simulink model "AC_motor_2_torque_control"  (R2024b)
settings: Solver=FixedStepAuto  StartTime=0.0  StopTime=Tsimulation  FixedStep=Ts  RelTol=1e-3
values from neighbouring files (symbols this model uses):
  J = 0.0226    [input_AIR80B4_2.m]    (also in input_AIR80B4_2_sc.m)
  Ki = 10    [input_AIR80B4_2.m]    (also in input_AIR80B4_2_sc.m)
  Kp = 10    [input_AIR80B4_2.m]    (also in input_AIR80B4_2_sc.m)
  P = 2    [input_AIR80B4_2.m]    (also in input_AIR80B4_2_sc.m)
  Rr = 1.274    [input_AIR80B4_2.m]    (also in input_AIR80B4_2_sc.m = Rr*((nturns_phase-fscnturns)/nturns_phase)^2)
  Rs = 3.523    [input_AIR80B4_2.m]    (also in input_AIR80B4_2_sc.m = Rs*((nturns_phase-fscnturns)/nturns_phase))
  Tlim = 11    [input_AIR80B4_2.m]    (also in input_AIR80B4_2_sc.m)
  Ts = 2e-5    (= 2e-05)    [input_AIR80B4_2.m]    (also in input_AIR80B4_2_sc.m)
  Tswrite = 0.24e-3    (= 0.00024)    [input_AIR80B4_2.m]    (also in input_AIR80B4_2_sc.m)
  Vdc = 460    [input_AIR80B4_2.m]    (also in input_AIR80B4_2_sc.m)
  wb = 2*pi*fb    (= 314.159265359)    [input_AIR80B4_2.m]    (also in input_AIR80B4_2_sc.m)
  Xlr = wb*Llr    (= 4.08407044967)    [input_AIR80B4_2.m]    (also in input_AIR80B4_2_sc.m)
  Xls = wb*Lls    (= 4.08407044967)    [input_AIR80B4_2.m]    (also in input_AIR80B4_2_sc.m)
  Xml = 1/(1/Xls+1/Xm+1/Xlr)    (= 2.00946288382)    [input_AIR80B4_2.m]    (also in input_AIR80B4_2_sc.m)
undefined symbols (not defined in the file or in its folder): DiscIntNeverNeededParam
libraries: simulink x2, spspowerguiLib x1
settings Model: Creator=rusla  LastModifiedBy=rusla

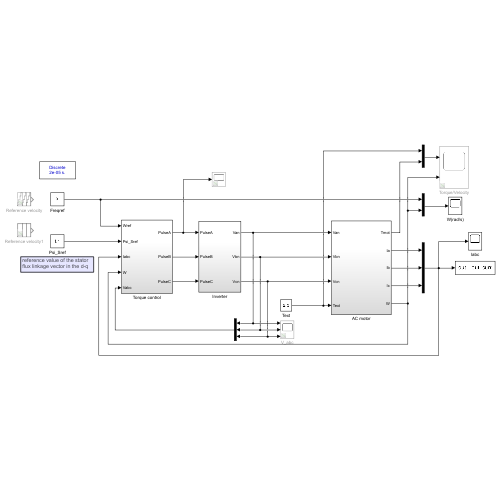
[thumbnail: Simulink's stored preview of the top-level diagram]
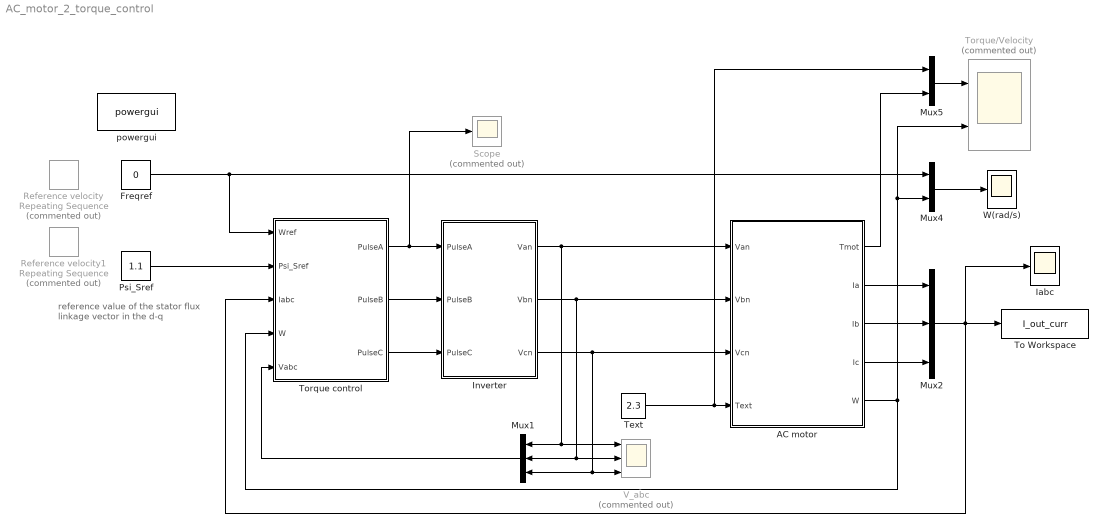
== system AC_motor_2_torque_control ==
  note: reference value of the stator
      | flux linkage vector in the d-q
  AC motor : Subsystem
  Freqref : Constant  Value=0
  Iabc : Scope
  Inverter : Subsystem
  Mux1 : Mux  Inputs=3
  Mux2 : Mux  Inputs=3
  Mux4 : Mux  Inputs=2
  Mux5 : Mux  Inputs=2
  Psi_Sref : Constant  Value=1.1
  Reference velocity : simulink/Sources/Repeating Sequence  Commented=on  rep_seq_t=[0 0.1 0.11 4 4.1 8 8.1 12 12.1 16]  rep_seq_y=[0 0 10 10 20 20 30 30 40 40]
  Reference velocity1 : simulink/Sources/Repeating Sequence  Commented=on  rep_seq_t=[0 0.1 0.11 10]  rep_seq_y=[0 0 2e-4 2e-4]
  Scope : Scope  Commented=on
  Text : Constant  Value=2.3
  To Workspace : ToWorkspace  VariableName=I_out_curr  SaveFormat=Structure With Time  SampleTime=Tswrite
  Torque control : Subsystem
  Torque/Velocity : Scope  Commented=on  NumInputPorts=2
  V_abc : Scope  Commented=on  NumInputPorts=3
  W(rad/s) : Scope
  powergui : spspowerguiLib/powergui  Priority=1  SimulationMode=Discrete  SampleTime=Ts  frequency=60  Iterations=50  frequencyindice=60  Pbase=100e6  ErrMax=1e-4  UnitsV=kV  UnitsW=MW  buscounter=0  FunctionMessages=off  echomessages=off  EnableUseOfTLC=off  CurrentSourceSwitches=off  DisableSnubberDevices=off  DisableRonSwitches=off  DisableVfSwitches=off  DisplayEquations=off  AutomaticDiscreteSolvers=off  SolverType=Tustin/Backward Euler (TBE)  Interpol=off  ExternalGateDelay=off  methode=off  Ts=100  x0status=blocks  SPID=on  SwTol=0  HookPort=off  NonlinearTolerance=1e-4  nMaxIteration=100  ContinueOnMaxIteration=off  RestoreLinks=warning  ResistiveCurrentMeasurement=off  Frange=[0:2:500]  Ylog=off  Xlog=on  ShowGrid=off  save=off  variable=ZData  structure=0  ZoomFFT=off  StartTime=0.0  cycles=1  DisplayStyle=1  fundamental=60  FreqAxis=off  MaxFrequency=1000  frequencyindicesteady=1  RmsSteady=1  display=off
  wires:
  Psi_Sref/1 -> Torque control/2(Psi_Sref)
  Freqref/1 -> Mux4/1, Torque control/1(Wref)
  Mux1/1 -> Torque control/5(Vabc)
  Inverter/1(Van) -> AC motor/1(Van), V_abc/1, Mux1/1
  Inverter/2(Vbn) -> AC motor/2(Vbn), V_abc/2, Mux1/2
  Inverter/3(Vcn) -> AC motor/3(Vcn), V_abc/3, Mux1/3
  Text/1 -> Mux5/1, AC motor/4(Text)
  Torque control/1(PulseA) -> Scope/1, Inverter/1(PulseA)
  Torque control/2(PulseB) -> Inverter/2(PulseB)
  Torque control/3(PulseC) -> Inverter/3(PulseC)
  AC motor/5(W) -> Torque control/4(W), Torque/Velocity/2, Mux4/2
  Mux2/1 -> To Workspace/1, Torque control/3(Iabc), Iabc/1
  AC motor/4(Ic) -> Mux2/3
  AC motor/3(Ib) -> Mux2/2
  AC motor/2(Ia) -> Mux2/1
  Mux4/1 -> W(rad/s)/1
  Mux5/1 -> Torque/Velocity/1
  AC motor/1(Tmot) -> Mux5/2

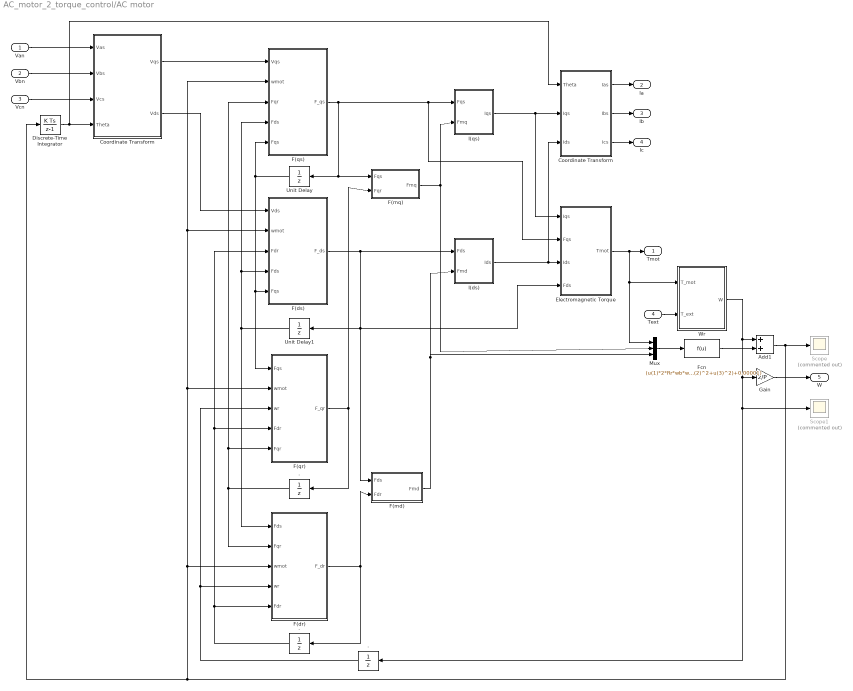
== system AC_motor_2_torque_control/AC motor ==
  Van : Inport
  Vbn : Inport  Port=2
  Vcn : Inport  Port=3
  Text : Inport  Port=4
  . : UnitDelay  SampleTime=Ts  HasFrameUpgradeWarning=on
  ". " : UnitDelay  SampleTime=Ts  HasFrameUpgradeWarning=on
  ".  " : UnitDelay  SampleTime=Ts  HasFrameUpgradeWarning=on
  Add1 : Sum
  Coordinate Transform : Subsystem
  "Coordinate Transform " : Subsystem
  Discrete-Time Integrator : DiscreteIntegrator  SampleTime=Ts  ICPrevOutput=DiscIntNeverNeededParam  ICPrevScaledInput=DiscIntNeverNeededParam
  Electromagnetic Torque : Subsystem
  F(dr) : Subsystem
  F(ds) : Subsystem
  F(md) : Subsystem
  F(mq) : Subsystem
  F(qr) : Subsystem
  F(qs) : Subsystem
  Fcn : Fcn  Expr=(u(1)*2*Rr*wb*wb)/(3*P*(u(2)^2+u(3)^2)+0.00001)
  Gain : Gain  Gain=2/P
  I(ds) : Subsystem
  I(qs) : Subsystem
  Mux : Mux  Inputs=3
  Scope : Scope  Commented=on
  Scope1 : Scope  Commented=on
  Unit Delay : UnitDelay  SampleTime=Ts  HasFrameUpgradeWarning=on
  Unit Delay1 : UnitDelay  SampleTime=Ts  HasFrameUpgradeWarning=on
  Wr : Subsystem
  Tmot : Outport
  Ia : Outport  Port=2
  Ib : Outport  Port=3
  Ic : Outport  Port=4
  W : Outport  Port=5
  wires:
  Gain/1 -> W/1
  Mux/1 -> Fcn/1
  Fcn/1 -> Add1/2
  F(md)/1(Fmd) -> I(ds)/2(Fmd), Mux/3
  ".  "/1 -> F(qr)/3(wr), F(dr)/4(wr)
  ". "/1 -> F(dr)/5(Fdr), F(qr)/4(Fdr), F(ds)/3(Fdr)
  ./1 -> F(dr)/2(Fqr), F(qs)/3(Fqr), F(qr)/5(Fqr)
  Unit Delay1/1 -> F(dr)/1(Fds), F(qs)/4(Fds), F(ds)/4(Fds)
  Unit Delay/1 -> F(qr)/1(Fqs), F(ds)/5(Fqs), F(qs)/5(Fqs)
  Add1/1 -> Scope/1, Discrete-Time Integrator/1, F(dr)/3(wmot), F(qr)/2(wmot), F(ds)/2(wmot), F(qs)/2("wmot ")
  Electromagnetic Torque/1(Tmot) -> Mux/1, Wr/1(T_mot), Tmot/1
  Text/1 -> Wr/2(T_ext)
  Discrete-Time Integrator/1 -> Coordinate Transform/1(Theta), "Coordinate Transform "/4(Theta)
  F(qs)/1(F_qs) -> Unit Delay/1, F(mq)/1(Fqs), I(qs)/1("Fqs "), Electromagnetic Torque/2(Fqs)
  F(qr)/1(F_qr) -> F(mq)/2(Fqr), ./1
  F(ds)/1(F_ds) -> Electromagnetic Torque/4(Fds), Unit Delay1/1, F(md)/1(Fds), I(ds)/1("Fds ")
  F(dr)/1(F_dr) -> F(md)/2(Fdr), ". "/1
  "Coordinate Transform "/1(Vqs) -> F(qs)/1(Vqs)
  Vbn/1 -> "Coordinate Transform "/2(Vbs)
  Vcn/1 -> "Coordinate Transform "/3(Vcs)
  "Coordinate Transform "/2(Vds) -> F(ds)/1(Vds)
  Van/1 -> "Coordinate Transform "/1(Vas)
  Wr/1(W) -> ".  "/1, Scope1/1, Gain/1, Add1/1
  I(qs)/1(Iqs) -> Coordinate Transform/2(Iqs), Electromagnetic Torque/1(Iqs)
  I(ds)/1(Ids) -> Coordinate Transform/3(Ids), Electromagnetic Torque/3(Ids)
  F(mq)/1(Fmq) -> Mux/2, I(qs)/2(Fmq)
  Coordinate Transform/1(Ias) -> Ia/1
  Coordinate Transform/2(Ibs) -> Ib/1
  Coordinate Transform/3(Ics) -> Ic/1

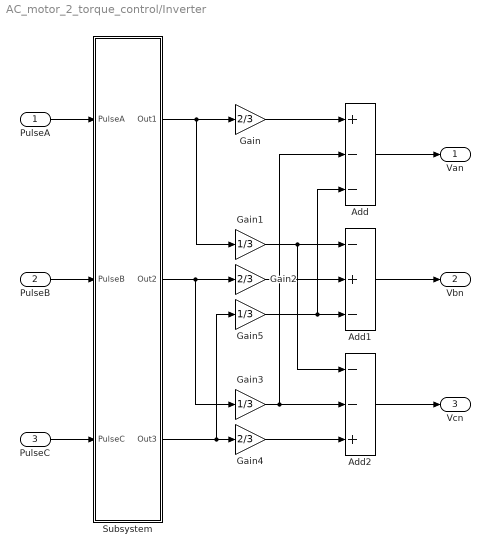
== system AC_motor_2_torque_control/Inverter ==
  PulseA : Inport
  PulseB : Inport  Port=2
  PulseC : Inport  Port=3
  Add : Sum  Inputs=+--
  Add1 : Sum  Inputs=-+-
  Add2 : Sum  Inputs=--+
  Gain : Gain  Gain=2/3
  Gain1 : Gain  Gain=1/3
  Gain2 : Gain  Gain=2/3
  Gain3 : Gain  Gain=1/3
  Gain4 : Gain  Gain=2/3
  Gain5 : Gain  Gain=1/3
  Subsystem : Subsystem
  Van : Outport
  Vbn : Outport  Port=2
  Vcn : Outport  Port=3
  wires:
  Gain1/1 -> Add1/1, Add2/1
  Gain2/1 -> Add1/2
  Gain/1 -> Add/1
  Gain5/1 -> Add1/3, Add/3
  Add1/1 -> Vbn/1
  Gain3/1 -> Add2/2, Add/2
  Add2/1 -> Vcn/1
  Add/1 -> Van/1
  Gain4/1 -> Add2/3
  Subsystem/1(Out1) -> Gain1/1, Gain/1
  Subsystem/3(Out3) -> Gain4/1, Gain5/1
  Subsystem/2(Out2) -> Gain3/1, Gain2/1
  PulseA/1 -> Subsystem/1(PulseA)
  PulseB/1 -> Subsystem/2(PulseB)
  PulseC/1 -> Subsystem/3(PulseC)

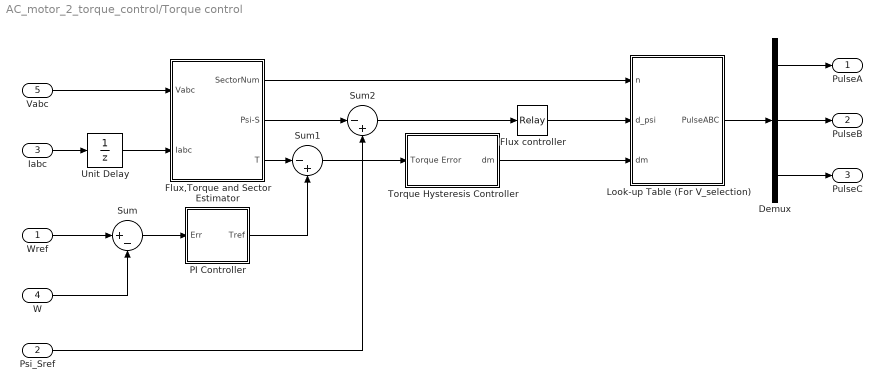
== system AC_motor_2_torque_control/Torque control ==
  Wref : Inport
  Psi_Sref : Inport  Port=2
  Iabc : Inport  Port=3
  W : Inport  Port=4
  Vabc : Inport  Port=5
  Demux : Demux  Outputs=3
  Flux controller : Relay  OnSwitchValue=0.02  OffSwitchValue=-0.02
  Flux,Torque and Sector Estimator : Subsystem
  Look-up Table (For V_selection) : MATLAB Function  TreatAsAtomicUnit=on
  PI Controller : Subsystem
  Sum : Sum  Inputs=|+-
  Sum1 : Sum  Inputs=|-+
  Sum2 : Sum  Inputs=|-+
  Torque Hysteresis Controller : Subsystem
  Unit Delay : UnitDelay  SampleTime=-1  HasFrameUpgradeWarning=on
  PulseA : Outport
  PulseB : Outport  Port=2
  PulseC : Outport  Port=3
  wires:
  Look-up Table (For V_selection)/1(PulseABC) -> Demux/1
  Vabc/1 -> Flux,Torque and Sector Estimator/1(Vabc)
  Demux/2 -> PulseB/1
  Demux/1 -> PulseA/1
  Unit Delay/1 -> Flux,Torque and Sector Estimator/2(Iabc)
  Demux/3 -> PulseC/1
  Wref/1 -> Sum/1
  Flux,Torque and Sector Estimator/3(T) -> Sum1/1
  Iabc/1 -> Unit Delay/1
  Sum1/1 -> Torque Hysteresis Controller/1(Torque Error)
  Sum/1 -> PI Controller/1(Err)
  Psi_Sref/1 -> Sum2/2
  Torque Hysteresis Controller/1(dm) -> Look-up Table (For V_selection)/3(dm)
  W/1 -> Sum/2
  Flux,Torque and Sector Estimator/1(SectorNum) -> Look-up Table (For V_selection)/1(n)
  Sum2/1 -> Flux controller/1
  Flux,Torque and Sector Estimator/2(Psi-S) -> Sum2/1
  Flux controller/1 -> Look-up Table (For V_selection)/2(d_psi)
  PI Controller/1(Tref) -> Sum1/2

== system AC_motor_2_torque_control/AC motor/Coordinate Transform ==
  Theta : Inport
  Iqs : Inport  Port=2
  Ids : Inport  Port=3
  Inverse Clark Transform : Subsystem
  Inverse Park Transform : Subsystem
  Ias : Outport
  Ibs : Outport  Port=2
  Ics : Outport  Port=3
  wires:
  Ids/1 -> Inverse Park Transform/2(Ids)
  Inverse Park Transform/2(I(qss)) -> Inverse Clark Transform/2(Iqss)
  Iqs/1 -> Inverse Park Transform/3(Iqs)
  Theta/1 -> Inverse Park Transform/1(Theta)
  Inverse Park Transform/1(I(dss)) -> Inverse Clark Transform/1(Idss)
  Inverse Clark Transform/2(Ibs) -> Ibs/1
  Inverse Clark Transform/1(Ias) -> Ias/1
  Inverse Clark Transform/3(Ics) -> Ics/1

== system AC_motor_2_torque_control/AC motor/Coordinate Transform  ==
  Vas : Inport
  Vbs : Inport  Port=2
  Vcs : Inport  Port=3
  Theta : Inport  Port=4
  Clark transform (betta inverted) 3 phase to 2 phase : Subsystem
  Park transform : Subsystem
  Vqs : Outport
  Vds : Outport  Port=2
  wires:
  Clark transform (betta inverted) 3 phase to 2 phase/1(Valpha) -> Park transform/1(Valpha)
  Clark transform (betta inverted) 3 phase to 2 phase/2(Vbetta) -> Park transform/2(Vbetta)
  Park transform/2("Vqs ") -> Vqs/1
  Theta/1 -> Park transform/3("Theta( e) (in rad.) ")
  Park transform/1(Vds) -> Vds/1
  Vbs/1 -> Clark transform (betta inverted) 3 phase to 2 phase/2(Vbs)
  Vcs/1 -> Clark transform (betta inverted) 3 phase to 2 phase/3(Vcs)
  Vas/1 -> Clark transform (betta inverted) 3 phase to 2 phase/1(Vas)

== system AC_motor_2_torque_control/AC motor/Electromagnetic Torque ==
  Iqs : Inport
  Fqs : Inport  Port=2
  Ids : Inport  Port=3
  Fds : Inport  Port=4
  Add : Sum  Inputs=+-
  Gain : Gain  Gain=(3*P)/(4*wb)
  Product : Product
  Product1 : Product
  Tmot : Outport
  wires:
  Product1/1 -> Add/2
  Add/1 -> Gain/1
  Product/1 -> Add/1
  Iqs/1 -> Product/2
  Ids/1 -> Product1/2
  Fqs/1 -> Product1/1
  Fds/1 -> Product/1
  Gain/1 -> Tmot/1

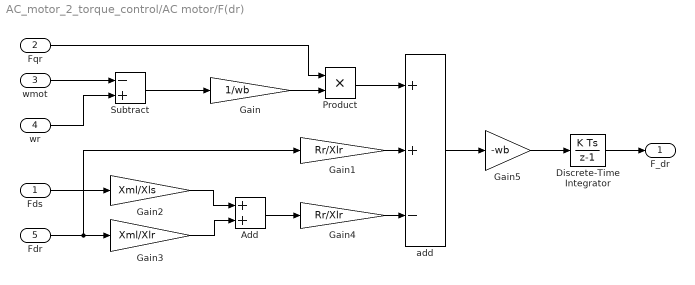
== system AC_motor_2_torque_control/AC motor/F(dr) ==
  Fds : Inport
  Fqr : Inport  Port=2
  wmot : Inport  Port=3
  wr : Inport  Port=4
  Fdr : Inport  Port=5
  Add : Sum
  Discrete-Time Integrator : DiscreteIntegrator  SampleTime=Ts  ICPrevOutput=DiscIntNeverNeededParam  ICPrevScaledInput=DiscIntNeverNeededParam
  Gain : Gain  Gain=1/wb
  Gain1 : Gain  Gain=Rr/Xlr
  Gain2 : Gain  Gain=Xml/Xls
  Gain3 : Gain  Gain=Xml/Xlr
  Gain4 : Gain  Gain=Rr/Xlr
  Gain5 : Gain  Gain=-wb
  Product : Product
  Subtract : Sum  Inputs=-+
  add : Sum  Inputs=++-
  F_dr : Outport
  wires:
  Product/1 -> add/1
  Fqr/1 -> Product/1
  Fdr/1 -> Gain1/1, Gain3/1
  Gain4/1 -> add/3
  Gain1/1 -> add/2
  wr/1 -> Subtract/2
  Gain/1 -> Product/2
  Gain3/1 -> Add/2
  Gain2/1 -> Add/1
  Fds/1 -> Gain2/1
  Add/1 -> Gain4/1
  Subtract/1 -> Gain/1
  wmot/1 -> Subtract/1
  add/1 -> Gain5/1
  Gain5/1 -> Discrete-Time Integrator/1
  Discrete-Time Integrator/1 -> F_dr/1

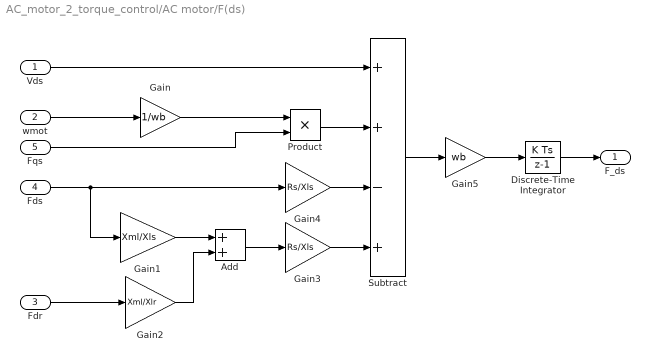
== system AC_motor_2_torque_control/AC motor/F(ds) ==
  Vds : Inport
  wmot : Inport  Port=2
  Fdr : Inport  Port=3
  Fds : Inport  Port=4
  Fqs : Inport  Port=5
  Add : Sum
  Discrete-Time Integrator : DiscreteIntegrator  SampleTime=Ts  ICPrevOutput=DiscIntNeverNeededParam  ICPrevScaledInput=DiscIntNeverNeededParam
  Gain : Gain  Gain=1/wb
  Gain1 : Gain  Gain=Xml/Xls
  Gain2 : Gain  Gain=Xml/Xlr
  Gain3 : Gain  Gain=Rs/Xls
  Gain4 : Gain  Gain=Rs/Xls
  Gain5 : Gain  Gain=wb
  Product : Product
  Subtract : Sum  Inputs=++-+
  F_ds : Outport
  wires:
  wmot/1 -> Gain/1
  Fdr/1 -> Gain2/1
  Gain1/1 -> Add/1
  Fds/1 -> Gain1/1, Gain4/1
  Gain4/1 -> Subtract/3
  Gain3/1 -> Subtract/4
  Add/1 -> Gain3/1
  Fqs/1 -> Product/2
  Product/1 -> Subtract/2
  Gain5/1 -> Discrete-Time Integrator/1
  Subtract/1 -> Gain5/1
  Discrete-Time Integrator/1 -> F_ds/1
  Gain2/1 -> Add/2
  Vds/1 -> Subtract/1
  Gain/1 -> Product/1

== system AC_motor_2_torque_control/AC motor/F(md) ==
  Fds : Inport
  Fdr : Inport  Port=2
  Add : Sum
  Gain1 : Gain  Gain=Xml/Xls
  Gain2 : Gain  Gain=Xml/Xlr
  Fmd : Outport
  wires:
  Gain1/1 -> Add/1
  Gain2/1 -> Add/2
  Fdr/1 -> Gain2/1
  Fds/1 -> Gain1/1
  Add/1 -> Fmd/1

== system AC_motor_2_torque_control/AC motor/F(mq) ==
  Fqs : Inport
  Fqr : Inport  Port=2
  Add : Sum
  Gain1 : Gain  Gain=Xml/Xls
  Gain2 : Gain  Gain=Xml/Xlr
  Fmq : Outport
  wires:
  Add/1 -> Fmq/1
  Fqs/1 -> Gain1/1
  Fqr/1 -> Gain2/1
  Gain2/1 -> Add/2
  Gain1/1 -> Add/1

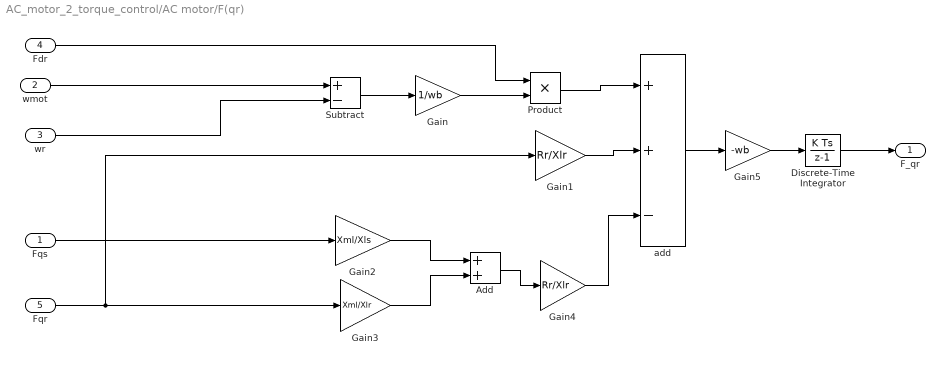
== system AC_motor_2_torque_control/AC motor/F(qr) ==
  Fqs : Inport
  wmot : Inport  Port=2
  wr : Inport  Port=3
  Fdr : Inport  Port=4
  Fqr : Inport  Port=5
  Add : Sum
  Discrete-Time Integrator : DiscreteIntegrator  SampleTime=Ts  ICPrevOutput=DiscIntNeverNeededParam  ICPrevScaledInput=DiscIntNeverNeededParam
  Gain : Gain  Gain=1/wb
  Gain1 : Gain  Gain=Rr/Xlr
  Gain2 : Gain  Gain=Xml/Xls
  Gain3 : Gain  Gain=Xml/Xlr
  Gain4 : Gain  Gain=Rr/Xlr
  Gain5 : Gain  Gain=-wb
  Product : Product
  Subtract : Sum  Inputs=+-
  add : Sum  Inputs=++-
  F_qr : Outport
  wires:
  Discrete-Time Integrator/1 -> F_qr/1
  Gain5/1 -> Discrete-Time Integrator/1
  add/1 -> Gain5/1
  wmot/1 -> Subtract/1
  Subtract/1 -> Gain/1
  Add/1 -> Gain4/1
  Fqs/1 -> Gain2/1
  Gain2/1 -> Add/1
  Gain3/1 -> Add/2
  Gain/1 -> Product/2
  wr/1 -> Subtract/2
  Gain1/1 -> add/2
  Gain4/1 -> add/3
  Fqr/1 -> Gain3/1, Gain1/1
  Fdr/1 -> Product/1
  Product/1 -> add/1

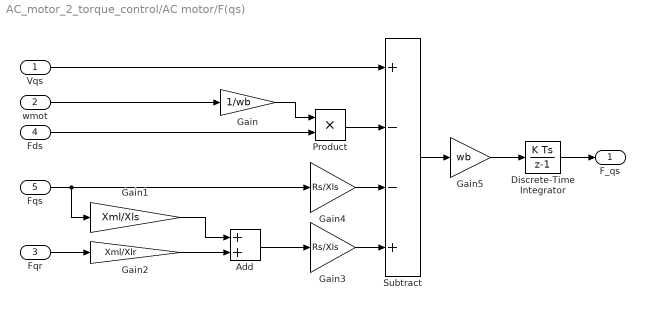
== system AC_motor_2_torque_control/AC motor/F(qs) ==
  Vqs : Inport
  "wmot " : Inport  Port=2
  Fqr : Inport  Port=3
  Fds : Inport  Port=4
  Fqs : Inport  Port=5
  Add : Sum
  Discrete-Time Integrator : DiscreteIntegrator  SampleTime=Ts  ICPrevOutput=DiscIntNeverNeededParam  ICPrevScaledInput=DiscIntNeverNeededParam
  Gain : Gain  Gain=1/wb
  Gain1 : Gain  Gain=Xml/Xls
  Gain2 : Gain  Gain=Xml/Xlr
  Gain3 : Gain  Gain=Rs/Xls
  Gain4 : Gain  Gain=Rs/Xls
  Gain5 : Gain  Gain=wb
  Product : Product
  Subtract : Sum  Inputs=+--+
  F_qs : Outport
  wires:
  Gain/1 -> Product/1
  Vqs/1 -> Subtract/1
  Gain2/1 -> Add/2
  Discrete-Time Integrator/1 -> F_qs/1
  Subtract/1 -> Gain5/1
  Gain5/1 -> Discrete-Time Integrator/1
  Product/1 -> Subtract/2
  Fds/1 -> Product/2
  Add/1 -> Gain3/1
  Gain3/1 -> Subtract/4
  Gain4/1 -> Subtract/3
  Fqs/1 -> Gain1/1, Gain4/1
  Gain1/1 -> Add/1
  Fqr/1 -> Gain2/1
  "wmot "/1 -> Gain/1

== system AC_motor_2_torque_control/AC motor/I(ds) ==
  "Fds " : Inport
  Fmd : Inport  Port=2
  Gain : Gain  Gain=1/Xls
  Subtract : Sum  Inputs=+-
  Ids : Outport
  wires:
  Fmd/1 -> Subtract/2
  "Fds "/1 -> Subtract/1
  Subtract/1 -> Gain/1
  Gain/1 -> Ids/1

== system AC_motor_2_torque_control/AC motor/I(qs) ==
  "Fqs " : Inport
  Fmq : Inport  Port=2
  Gain : Gain  Gain=1/Xls
  Subtract : Sum  Inputs=+-
  Iqs : Outport
  wires:
  Gain/1 -> Iqs/1
  Subtract/1 -> Gain/1
  "Fqs "/1 -> Subtract/1
  Fmq/1 -> Subtract/2

== system AC_motor_2_torque_control/AC motor/Wr ==
  T_mot : Inport
  T_ext : Inport  Port=2
  Add : Sum  Inputs=+-
  Discrete-Time Integrator : DiscreteIntegrator  gainval=Ktorquegain  SampleTime=Ts  ICPrevOutput=DiscIntNeverNeededParam  ICPrevScaledInput=DiscIntNeverNeededParam
  Gain : Gain  Gain=P/(2*J)
  W : Outport
  wires:
  T_mot/1 -> Add/1
  T_ext/1 -> Add/2
  Add/1 -> Gain/1
  Gain/1 -> Discrete-Time Integrator/1
  Discrete-Time Integrator/1 -> W/1

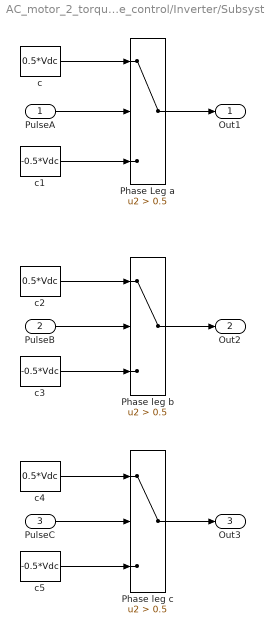
== system AC_motor_2_torque_control/Inverter/Subsystem ==
  PulseA : Inport
  PulseB : Inport  Port=2
  PulseC : Inport  Port=3
  Phase Leg a : Switch  Criteria=u2 > Threshold  Threshold=0.5  SaturateOnIntegerOverflow=off  InputSameDT=off
  Phase leg b : Switch  Criteria=u2 > Threshold  Threshold=0.5  SaturateOnIntegerOverflow=off  InputSameDT=off
  "Phase leg c " : Switch  Criteria=u2 > Threshold  Threshold=0.5  SaturateOnIntegerOverflow=off  InputSameDT=off
  c : Constant  Value=0.5*Vdc
  c1 : Constant  Value=-0.5*Vdc
  c2 : Constant  Value=0.5*Vdc
  c3 : Constant  Value=-0.5*Vdc
  c4 : Constant  Value=0.5*Vdc
  c5 : Constant  Value=-0.5*Vdc
  Out1 : Outport
  Out2 : Outport  Port=2
  Out3 : Outport  Port=3
  wires:
  "Phase leg c "/1 -> Out3/1
  c5/1 -> "Phase leg c "/3
  c3/1 -> Phase leg b/3
  c/1 -> Phase Leg a/1
  Phase Leg a/1 -> Out1/1
  Phase leg b/1 -> Out2/1
  c4/1 -> "Phase leg c "/1
  PulseB/1 -> Phase leg b/2
  PulseA/1 -> Phase Leg a/2
  PulseC/1 -> "Phase leg c "/2
  c1/1 -> Phase Leg a/3
  c2/1 -> Phase leg b/1

== system AC_motor_2_torque_control/Torque control/Flux,Torque and Sector Estimator ==
  Vabc : Inport
  Iabc : Inport  Port=2
  Flux and Torque Estimator : Subsystem
  Scope : Scope  Commented=on
  Sector Estimation : MATLAB Function  TreatAsAtomicUnit=on
  SectorNum : Outport
  Psi-S : Outport  Port=2
  T : Outport  Port=3
  wires:
  Iabc/1 -> Flux and Torque Estimator/2(Iabc)
  Vabc/1 -> Flux and Torque Estimator/1(V_abc)
  Flux and Torque Estimator/4(PsiBeta) -> Sector Estimation/2(PsiBeta)
  Flux and Torque Estimator/3(PsiAlpha) -> Sector Estimation/1(PsiAlpha)
  Sector Estimation/1(n) -> SectorNum/1
  Flux and Torque Estimator/1(Psi_S) -> Psi-S/1
  Flux and Torque Estimator/2(TransientTorque) -> T/1
  Sector Estimation/2(angl) -> Scope/1

== system AC_motor_2_torque_control/Torque control/PI Controller ==
  Err : Inport
  "Integrator " : DiscreteIntegrator  SampleTime=Ts  LimitOutput=on  UpperSaturationLimit=Tlim  LowerSaturationLimit=-Tlim  ICPrevOutput=DiscIntNeverNeededParam  ICPrevScaledInput=DiscIntNeverNeededParam
  Ki : Gain  Gain=Ki
  Kp : Gain  Gain=Kp
  Saturation : Saturate  UpperLimit=Tlim  LowerLimit=-Tlim
  Sum1 : Sum  Inputs=|++
  Tref : Outport
  wires:
  Saturation/1 -> Tref/1
  Sum1/1 -> Saturation/1
  "Integrator "/1 -> Sum1/2
  Kp/1 -> Sum1/1
  Ki/1 -> "Integrator "/1
  Err/1 -> Kp/1, Ki/1

== system AC_motor_2_torque_control/Torque control/Torque Hysteresis Controller ==
  Torque Error : Inport
  Add : Sum
  Flux controller1 : Relay  OnSwitchValue=0.2  OffSwitchValue=0
  Flux controller2 : Relay  OnSwitchValue=0  OffSwitchValue=-0.2  OnOutputValue=0  OffOutputValue=-1
  dm : Outport
  wires:
  Torque Error/1 -> Flux controller1/1, Flux controller2/1
  Flux controller1/1 -> Add/1
  Flux controller2/1 -> Add/2
  Add/1 -> dm/1

== system AC_motor_2_torque_control/AC motor/Coordinate Transform/Inverse Clark Transform ==
  Idss : Inport
  Iqss : Inport  Port=2
  Add : Sum
  Add1 : Sum
  Gain : Gain  Gain=-0.5
  Gain1 : Gain  Gain=-sqrt(3)/2
  Gain2 : Gain  Gain=-0.5
  Gain3 : Gain  Gain=sqrt(3)/2
  Ias : Outport
  Ibs : Outport  Port=2
  Ics : Outport  Port=3
  wires:
  Iqss/1 -> Gain/1, Ias/1, Gain2/1
  Idss/1 -> Gain1/1, Gain3/1
  Gain/1 -> Add/1
  Gain1/1 -> Add/2
  Add1/1 -> Ics/1
  Gain2/1 -> Add1/1
  Add/1 -> Ibs/1
  Gain3/1 -> Add1/2

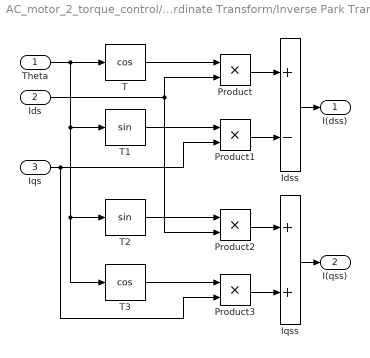
== system AC_motor_2_torque_control/AC motor/Coordinate Transform/Inverse Park Transform ==
  Theta : Inport
  Ids : Inport  Port=2
  Iqs : Inport  Port=3
  Idss : Sum  Inputs=+-
  Iqss : Sum
  Product{,1..3} (4 alike) : Product
  T : Trigonometry  Operator=cos
  T1 : Trigonometry
  T2 : Trigonometry
  T3 : Trigonometry  Operator=cos
  I(dss) : Outport
  I(qss) : Outport  Port=2
  wires:
  T3/1 -> Product3/1
  Product2/1 -> Iqss/1
  Ids/1 -> Product2/2, Product/2
  Theta/1 -> T1/1, T3/1, T2/1, T/1
  Product3/1 -> Iqss/2
  Iqs/1 -> Product3/2, Product1/2
  T2/1 -> Product2/1
  T1/1 -> Product1/1
  Iqss/1 -> I(qss)/1
  Idss/1 -> I(dss)/1
  Product1/1 -> Idss/2
  Product/1 -> Idss/1
  T/1 -> Product/1

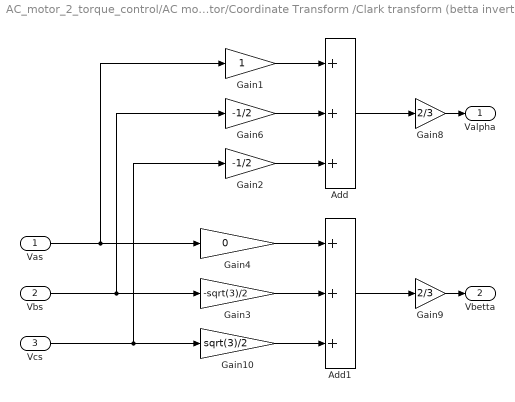
== system AC_motor_2_torque_control/AC motor/Coordinate Transform /Clark transform (betta inverted) 3 phase to 2 phase ==
  Vas : Inport
  Vbs : Inport  Port=2
  Vcs : Inport  Port=3
  Add : Sum  Inputs=+++
  Add1 : Sum  Inputs=+++
  Gain1 : Gain
  Gain10 : Gain  Gain=sqrt(3)/2
  Gain2 : Gain  Gain=-1/2
  Gain3 : Gain  Gain=-sqrt(3)/2
  Gain4 : Gain  Gain=0
  Gain6 : Gain  Gain=-1/2
  Gain8 : Gain  Gain=2/3
  Gain9 : Gain  Gain=2/3
  Valpha : Outport
  Vbetta : Outport  Port=2
  wires:
  Gain2/1 -> Add/3
  Gain9/1 -> Vbetta/1
  Gain8/1 -> Valpha/1
  Add1/1 -> Gain9/1
  Add/1 -> Gain8/1
  Gain6/1 -> Add/2
  Gain1/1 -> Add/1
  Gain4/1 -> Add1/1
  Gain3/1 -> Add1/2
  Vcs/1 -> Gain10/1, Gain2/1
  Gain10/1 -> Add1/3
  Vas/1 -> Gain4/1, Gain1/1
  Vbs/1 -> Gain6/1, Gain3/1

== system AC_motor_2_torque_control/AC motor/Coordinate Transform /Park transform ==
  Valpha : Inport
  Vbetta : Inport  Port=2
  "Theta( e) (in rad.) " : Inport  Port=3
  Add : Sum
  Add2 : Sum  Inputs=+-
  Product{,1..2,4} (4 alike) : Product
  t : Trigonometry  Operator=cos
  t1 : Trigonometry
  t2 : Trigonometry  Operator=cos
  t3 : Trigonometry
  Vds : Outport
  "Vqs " : Outport  Port=2
  wires:
  Valpha/1 -> Product4/1, Product1/1
  Product2/1 -> Add2/2
  t3/1 -> Product2/2
  Product4/1 -> Add2/1
  t2/1 -> Product4/2
  Product1/1 -> Add/2
  t1/1 -> Product1/2
  Product/1 -> Add/1
  Add2/1 -> "Vqs "/1
  Add/1 -> Vds/1
  "Theta( e) (in rad.) "/1 -> t3/1, t2/1, t/1, t1/1
  Vbetta/1 -> Product2/1, Product/1
  t/1 -> Product/2

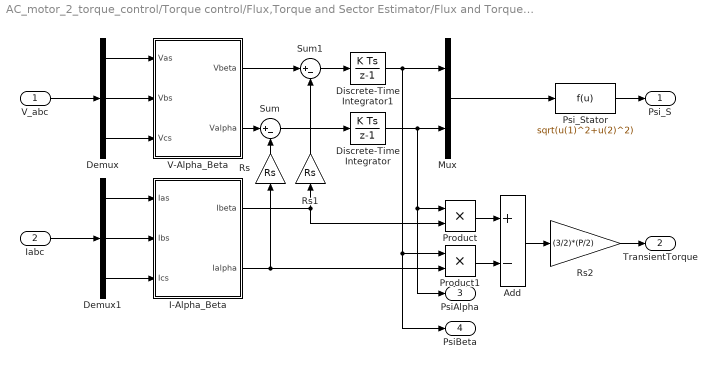
== system AC_motor_2_torque_control/Torque control/Flux,Torque and Sector Estimator/Flux and Torque Estimator ==
  V_abc : Inport
  Iabc : Inport  Port=2
  Add : Sum  Inputs=+-
  Demux : Demux  Outputs=3
  Demux1 : Demux  Outputs=3
  Discrete-Time Integrator : DiscreteIntegrator  SampleTime=Ts  ICPrevOutput=DiscIntNeverNeededParam  ICPrevScaledInput=DiscIntNeverNeededParam
  Discrete-Time Integrator1 : DiscreteIntegrator  SampleTime=Ts  ICPrevOutput=DiscIntNeverNeededParam  ICPrevScaledInput=DiscIntNeverNeededParam
  I-Alpha_Beta : Subsystem
  Mux : Mux  Inputs=2
  Product : Product
  Product1 : Product
  Psi_Stator : Fcn  Expr=sqrt(u(1)^2+u(2)^2)
  Rs : Gain  Gain=Rs
  Rs1 : Gain  Gain=Rs
  Rs2 : Gain  Gain=(3/2)*(P/2)
  Sum : Sum  Inputs=|+-
  Sum1 : Sum  Inputs=|+-
  V-Alpha_Beta : Subsystem
  Psi_S : Outport
  TransientTorque : Outport  Port=2
  PsiAlpha : Outport  Port=3
  PsiBeta : Outport  Port=4
  wires:
  Discrete-Time Integrator1/1 -> PsiBeta/1, Product1/1, Mux/1
  Rs2/1 -> TransientTorque/1
  Psi_Stator/1 -> Psi_S/1
  Add/1 -> Rs2/1
  Product1/1 -> Add/2
  Product/1 -> Add/1
  Discrete-Time Integrator/1 -> Product/1, PsiAlpha/1, Mux/2
  Mux/1 -> Psi_Stator/1
  Sum1/1 -> Discrete-Time Integrator1/1
  Rs1/1 -> Sum1/2
  Sum/1 -> Discrete-Time Integrator/1
  Rs/1 -> Sum/2
  Demux/2 -> V-Alpha_Beta/2(Vbs)
  Demux/1 -> V-Alpha_Beta/1(Vas)
  V_abc/1 -> Demux/1
  Demux/3 -> V-Alpha_Beta/3(Vcs)
  I-Alpha_Beta/2(Ialpha) -> Rs/1, Product1/2
  I-Alpha_Beta/1(Ibeta) -> Rs1/1, Product/2
  V-Alpha_Beta/1(Vbeta) -> Sum1/1
  V-Alpha_Beta/2(Valpha) -> Sum/1
  Demux1/2 -> I-Alpha_Beta/2(Ibs)
  Demux1/3 -> I-Alpha_Beta/3(Ics)
  Demux1/1 -> I-Alpha_Beta/1(Ias)
  Iabc/1 -> Demux1/1

== system AC_motor_2_torque_control/Torque control/Flux,Torque and Sector Estimator/Flux and Torque Estimator/I-Alpha_Beta ==
  Ias : Inport
  Ibs : Inport  Port=2
  Ics : Inport  Port=3
  Add : Sum  Inputs=+++
  Add1 : Sum  Inputs=+++
  Gain : Gain  Gain=0
  Gain1 : Gain  Gain=sqrt(3)/2
  Gain2 : Gain  Gain=-sqrt(3)/2
  Gain3 : Gain
  Gain4 : Gain  Gain=-1/2
  Gain5 : Gain  Gain=-1/2
  Gain8 : Gain  Gain=2/3
  Gain9 : Gain  Gain=2/3
  Ibeta : Outport
  Ialpha : Outport  Port=2
  wires:
  Ibs/1 -> Gain1/1, Gain4/1
  Ias/1 -> Gain/1, Gain3/1
  Gain5/1 -> Add1/3
  Ics/1 -> Gain5/1, Gain2/1
  Gain4/1 -> Add1/2
  Gain3/1 -> Add1/1
  Gain/1 -> Add/1
  Gain1/1 -> Add/2
  Add/1 -> Gain8/1
  Add1/1 -> Gain9/1
  Gain8/1 -> Ibeta/1
  Gain9/1 -> Ialpha/1
  Gain2/1 -> Add/3

== system AC_motor_2_torque_control/Torque control/Flux,Torque and Sector Estimator/Flux and Torque Estimator/V-Alpha_Beta ==
  Vas : Inport
  Vbs : Inport  Port=2
  Vcs : Inport  Port=3
  Add : Sum  Inputs=+++
  Add1 : Sum  Inputs=+++
  Gain : Gain  Gain=0
  Gain1 : Gain  Gain=sqrt(3)/2
  Gain2 : Gain  Gain=-sqrt(3)/2
  Gain3 : Gain
  Gain4 : Gain  Gain=-1/2
  Gain5 : Gain  Gain=-1/2
  Gain8 : Gain  Gain=2/3
  Gain9 : Gain  Gain=2/3
  Vbeta : Outport
  Valpha : Outport  Port=2
  wires:
  Gain2/1 -> Add/3
  Gain9/1 -> Valpha/1
  Gain8/1 -> Vbeta/1
  Add1/1 -> Gain9/1
  Add/1 -> Gain8/1
  Gain1/1 -> Add/2
  Gain/1 -> Add/1
  Gain3/1 -> Add1/1
  Gain4/1 -> Add1/2
  Vcs/1 -> Gain5/1, Gain2/1
  Gain5/1 -> Add1/3
  Vas/1 -> Gain/1, Gain3/1
  Vbs/1 -> Gain1/1, Gain4/1

== matlab function AC_motor_2_torque_control/Torque control/Look-up Table (For V_selection) ==
  data: n input; d_psi input; PulseABC output; dm input
function PulseABC=V_selection(n,d_psi,dm)
v=0;
%SECTOR 1 :
if(n==1)&&(d_psi==1)&&(dm==1)
    v=2;
elseif(n==1)&&(d_psi==1)&&(dm==0)
    v=7;
elseif(n==1)&&(d_psi==1)&&(dm==-1)
    v=6;
elseif(n==1)&&(d_psi==0)&&(dm==1)
    v=3;
elseif(n==1)&&(d_psi==0)&&(dm==0)
    v=0;
elseif(n==1)&&(d_psi==0)&&(dm==-1)
    v=5;
%SECTOR 2 :
elseif(n==2)&&(d_psi==1)&&(dm==1)
    v=3;
elseif(n==2)&&(d_psi==1)&&(dm==0)
    v=0;
elseif(n==2)&&(d_psi==1)&&(dm==-1)
    v=1;
elseif(n==2)&&(d_psi==0)&&(dm==1)
    v=4;
elseif(n==2)&&(d_psi==0)&&(dm==0)
    v=7;
elseif(n==2)&&(d_psi==0)&&(dm==-1)
    v=6;
%SECTOR 3 :
elseif(n==3)&&(d_psi==1)&&(dm==1)
    v=4;
elseif(n==3)&&(d_psi==1)&&(dm==0)
    v=7;
elseif(n==3)&&(d_psi==1)&&(dm==-1)
    v=2;
elseif(n==3)&&(d_psi==0)&&(dm==1)
    v=5;
elseif(n==3)&&(d_psi==0)&&(dm==0)
    v=0;
elseif(n==3)&&(d_psi==0)&&(dm==-1)
    v=1;
%SECTOR 4 :
elseif(n==4)&&(d_psi==1)&&(dm==1)
    v=5;
elseif(n==4)&&(d_psi==1)&&(dm==0)
    v=0;
elseif(n==4)&&(d_psi==1)&&(dm==-1)
    v=3;
elseif(n==4)&&(d_psi==0)&&(dm==1)
    v=6;
elseif(n==4)&&(d_psi==0)&&(dm==0)
    v=7;
elseif(n==4)&&(d_psi==0)&&(dm==-1)
    v=2;
%SECTOR 5 :
elseif(n==5)&&(d_psi==1)&&(dm==1)
    v=6;
elseif(n==5)&&(d_psi==1)&&(dm==0)
    v=7;
elseif(n==5)&&(d_psi==1)&&(dm==-1)
    v=4;
elseif(n==5)&&(d_psi==0)&&(dm==1)
    v=1;
elseif(n==5)&&(d_psi==0)&&(dm==0)
    v=0;
elseif(n==5)&&(d_psi==0)&&(dm==-1)
    v=3;
%SECTOR 6 :
elseif(n==6)&&(d_psi==1)&&(dm==1)
    v=1;
elseif(n==6)&&(d_psi==1)&&(dm==0)
    v=0;
elseif(n==6)&&(d_psi==1)&&(dm==-1)
    v=5;
elseif(n==6)&&(d_psi==0)&&(dm==1)
    v=2;
elseif(n==6)&&(d_psi==0)&&(dm==0)
    v=7;
elseif(n==6)&&(d_psi==0)&&(dm==-1)
    v=4;
end
switch v
    case 0
        PulseABC = [0 0 0];
    case 1
        PulseABC = [1 0 0];
    case 2
        PulseABC = [1 1 0];
    case 3
        PulseABC = [0 1 0];
    case 4
        PulseABC = [0 1 1];
    case 5
        PulseABC = [0 0 1];
    case 6
        PulseABC = [1 0 1];
    otherwise
        PulseABC = [1 1 1];
end

== matlab function AC_motor_2_torque_control/Torque control/Flux,Torque and Sector Estimator/Sector Estimation ==
  data: PsiAlpha input; n output; PsiBeta input; angl output
function [n,angl]=SECTOR(PsiAlpha,PsiBeta)
n=0;
angl=atan2(PsiBeta,PsiAlpha);
if(angl>=-pi/6)&&(angl<pi/6)
    n=1;
elseif(angl>=pi/6)&&(angl<pi/2)
    n=2;
elseif(angl>=pi/2)&&(angl<5*pi/6)
    n=3;
elseif(angl>=5*pi/6)&&(angl<pi)
    n=4;
elseif(angl>=-pi)&&(angl<-5*pi/6)
    n=4;
elseif(angl>=-5*pi/6)&&(angl<-pi/2)
    n=5;
elseif(angl>=-pi/2)&&(angl<-pi/6)
    n=6;
end
angl = angl*180/pi;
